simulink model "Load_Flow_V2"  (R2024a)
settings: Solver=ode23tb  StartTime=0.0  StopTime=0.3  RelTol=1e-4
undefined symbols (not defined in the file): Acid, D1, Delta, Lead
libraries: spsGroundLib x7, spsVoltageMeasurementLib x7, spsFourierLib x6, simulink x6, spsThreePhaseBreakerLib x4, spsThreePhaseTransformerTwoWindingsLib x3, spsThreePhaseParallelRLCLoadLib x3, spsThreePhaseSourceLib x2, spsThreePhaseFaultLib x2, spsBatteryLib x1, spsCurrentMeasurementLib x1, spsSeriesRLCBranchLib x1
settings Model: Creator=Sindid  LastModifiedBy=sindi
settings DataIOCC: SaveOutput=off

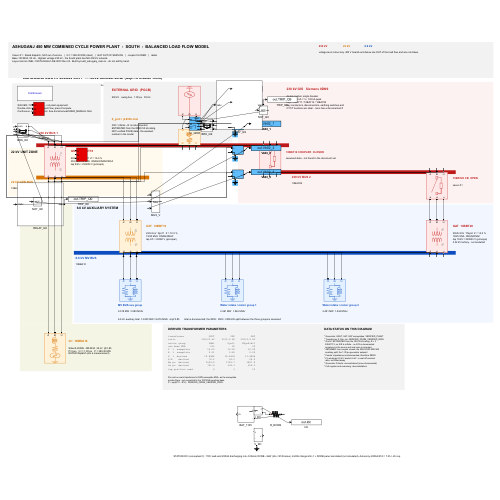
[thumbnail: Simulink's stored preview of the top-level diagram]
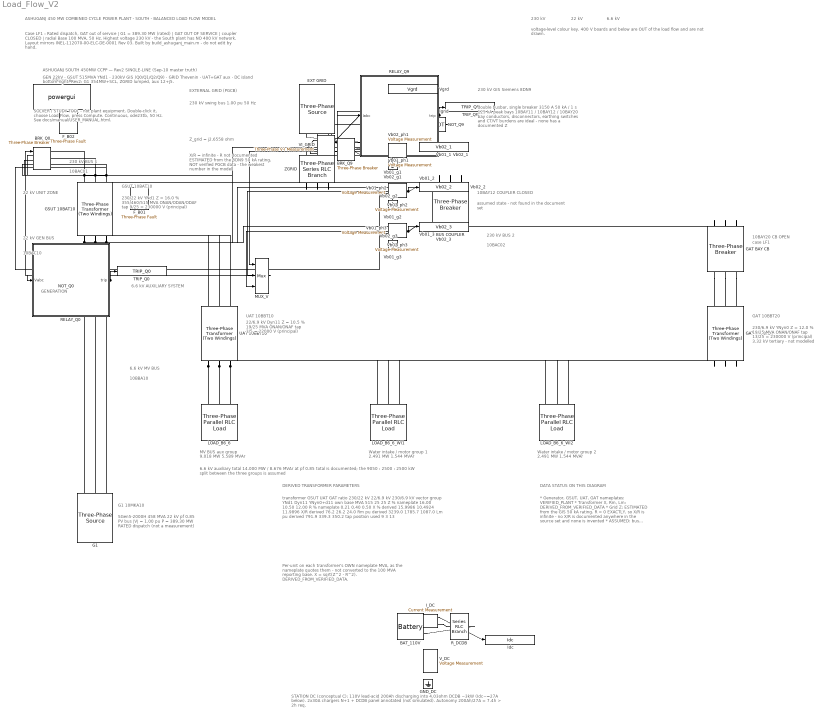
== system Load_Flow_V2 ==
  note: EXTERNAL GRID (PGCB)
  note: 230 kV swing bus 1.00 pu 50 Hz
  note: Z_grid = j2.6558 ohm
  note: X/R = infinite - R not documented
      | ESTIMATED from the 8DN9 50 kA rating,
      | NOT verified PGCB data - the weakest
      | number in the model
  note: GSUT 10BAT10
  note: 230/22 kV  YNd1  Z = 16.0 %
      | 355/460/515 MVA  ONAN/ODAN/ODAF
      | tap 9/25 = 230000 V (principal)
  note: 230 kV GIS Siemens 8DN9
  note: double busbar, single breaker
      | 3150 A  50 kA / 1 s  125 kA peak
      | bays 10BAY11 / 10BAY12 / 10BAY20
      | bay conductors, disconnectors, earthing switches and
      | CT/VT burdens are ideal - none has a documented Z
  note: 10BAY12 COUPLER CLOSED
  note: assumed state - not found in the document set
  note: 10BAY20 CB OPEN
  note: case LF1
  note: G1 10MKA10
  note: SGen5-2000H  458 MVA  22 kV  pf 0.85
      | PV bus   |V| = 1.00 pu   P = 389.30 MW
      | RATED dispatch (not a measurement)
  note: MV BUS aux group
  note: 9.018 MW 5.589 MVAr
  note: Water intake / motor group 1
  note: 2.491 MW 1.544 MVAr
  note: Water intake / motor group 2
  note: 2.491 MW 1.544 MVAr
  note: UAT 10BBT10
  note: 22/6.9 kV  Dyn11  Z = 10.5 %
      | 19/25 MVA  ONAN/ONAF
      | tap 3/5 = 22000 V (principal)
  note: GAT 10BBT20
  note: 230/6.9 kV  YNyn0  Z = 12.0 %
      | 19/25 MVA  ONAN/ONAF
      | tap 13/25 = 230000 V (principal)
      | 3.32 kV tertiary - not modelled
  note: 6.6 kV auxiliary total 14.000 MW / 8.676 MVAr at pf 0.85 total is documented; the 9050 : 2500 : 2500 kW split between the three groups is assumed
  note: 230 kV BUS 1
  note: 10BAC01
  note: 230 kV BUS 2
  note: 10BAC02
  note: 22 kV GEN BUS
  note: 10BAC10
  note: 6.6 kV MV BUS
  note: 10BBA10
  note: 22 kV UNIT ZONE
  note: 6.6 kV AUXILIARY SYSTEM
  note: GENERATION
  note: ASHUGANJ 450 MW COMBINED CYCLE POWER PLANT - SOUTH - BALANCED LOAD FLOW MODEL
  note: Case LF1 : Rated dispatch, GAT out of service   |   G1 = 389.30 MW (rated)   |   GAT OUT OF SERVICE   |   coupler CLOSED   |   radial
      | Base 100 MVA, 50 Hz.  Highest voltage 230 kV - the South plant has NO 400 kV network.
      | Layout mirrors INEL-112070-00-ELC-DE-0001 Rev 03.  Built by build_ashuganj_main.m - do not edit by hand.
  note: 230 kV
  note: 22 kV
  note: 6.6 kV
  note: voltage-level colour key. 400 V boards and below are OUT of the load flow and are not drawn.
  note: SOLVER / STUDY TOOL - not plant equipment.
      | Double-click it, choose Load Flow, press Compute.
      | Continuous, ode23tb, 50 Hz. See docs/manual/USER_MANUAL.html.
  note: DERIVED TRANSFORMER PARAMETERS
  note: transformer                 GSUT           UAT           GAT
      | ratio                  230/22 kV     22/6.9 kV    230/6.9 kV
      | vector group                YNd1         Dyn11     YNyn0+d11
      | own base MVA                 515            25            25
      | Z  %  nameplate            16.00         10.50         12.00
      | R  %  nameplate             0.21          0.40          0.50
      | X  %  derived            15.9986       10.4924       11.9896
      | X/R    derived              76.2          26.2          24.0
      | Rm pu  derived            3239.0        1785.7        1087.0
      | Lm pu  derived             791.9         339.3         350.2
      | tap position used              9             3            13
  note: Per-unit on each transformer's OWN nameplate MVA, as the nameplate
      | quotes them - not converted to the 100 MVA reporting base.
      | X = sqrt(Z^2 - R^2).  DERIVED_FROM_VERIFIED_DATA.
  note: DATA STATUS ON THIS DIAGRAM
  note: * Generator, GSUT, UAT, GAT nameplates: VERIFIED_PLANT
      | * Transformer X, Rm, Lm: DERIVED_FROM_VERIFIED_DATA
      | * Grid Z: ESTIMATED from the GIS 50 kA rating. R = 0
      |   EXACTLY, so X/R is infinite - no X/R is documented
      |   anywhere in the source set and none is invented
      | * ASSUMED: bus coupler closed, the 9050:2500:2500 kW
      |   auxiliary split, the 1.00 pu generator setpoint
      | * Feeder impedances undocumented, therefore ZERO
      | * LV windings 6.9 kV, loads 6.6 kV - a real off-nominal
      |   ratio, not tidied away
      | * Generator Q limits: unconstrained (none documented)
      | * Full register and reasoning: docs/validation/
  note: ASHUGANJ SOUTH 450MW CCPP — Rev2 SINGLE-LINE (Sep-10 master truth)
  note: GEN 22kV · GSUT 515MVA YNd1 · 230kV GIS (Q0/Q1/Q2/Q9) · GRID Thevenin · UAT+GAT aux · DC island bottom-right. Rev2: G1 354MW+SCL, ZGRID lumped, aux 12+j5.
  note: STATION DC (conceptual C): 110V lead-acid 200Ah discharging into 4.03ohm DCDB ~3kW (Idc~=27A below). 2x30A chargers N+1 + DCDB panel annotated (not simulated). Autonomy 200Ah/27A = 7.4h > 2h req.
  BAT_110V : spsBatteryLib/Battery  BatType=Lead-Acid  ShowTempParam=off  ThermalPreset=no  ShowAgeParam=off  NomV=110  NomQ=200  SOC=100  Batt_Tr=30  PresetModel=on  MaxQ=208.3333  MinV=82.5  FullV=119.7697  Dis_rate=40  R=0.0055  Normal_OP=62.0556  expZone="[111.9901     0.6666667]"  current=[6.5 13 32.5]  Units=Time  Tci=20  NomT=20  T2=-30  MaxQ2=4.8  FullV2=7.1  Normal_OP2=5.655  expZone2="[6.58           1]"  Rca=0.6  ti=2000  Dp=0  Neq0=0  Tsim=1e6  Ta1=25  Qeol=5.4*0.9  Reol=0.013333*1.2  Char_age=[2.3478, 3]  Dis_age=[2.3478, 10]  N1=1500  N2=10500  N3=1000  N4=1400  Ta2=45  N5=950
  BRK_Q0 : spsThreePhaseBreakerLib/Three-Phase Breaker  InitialState=closed  SwitchA=on  SwitchB=on  SwitchC=on  SwitchTimes="[1/60  5/60]"  External=on  BreakerResistance=0.01  SnubberResistance=1e6  SnubberCapacitance=inf  Measurements=None
  BRK_Q9 : spsThreePhaseBreakerLib/Three-Phase Breaker  InitialState=closed  SwitchA=on  SwitchB=on  SwitchC=on  SwitchTimes="[1/60  5/60]"  External=on  BreakerResistance=0.01  SnubberResistance=1e6  SnubberCapacitance=inf  Measurements=None
  BUS COUPLER : spsThreePhaseBreakerLib/Three-Phase Breaker  InitialState=closed  SwitchA=on  SwitchB=on  SwitchC=on  SwitchTimes=[1e6]  External=off  BreakerResistance=0.01  SnubberResistance=1e6  SnubberCapacitance=inf  Measurements=None
  EXT GRID : spsThreePhaseSourceLib/Three-Phase Source  InternalConnection=Yg  VoltagePhases=off  Voltage=230000  PhaseAngle=0  Voltage_phases=[25e3 25e3 25e3]/sqrt(3)  PhaseAngles_phases=[0 -120 +120]  Frequency=50  NonIdealSource=off  SpecifyImpedance=off  Resistance=0.8929  Inductance=16.58e-3  ShortCircuitLevel=100e6  BaseVoltage=230000  XRratio=7  BusType=swing  Pref=10e3  Qref=0  Prefabc=[10e3, 10e3, 10e3]  Qrefabc=[0, 0, 0]  Qmin=-inf  Qmax=inf
  F_B01 : spsThreePhaseFaultLib/Three-Phase Fault  InitialStates=0  FaultA=off  FaultB=off  FaultC=off  GroundFault=off  SwitchTimes=[0.05]  External=off  SwitchStatus=NaN  FaultResistance=1e-4  GroundResistance=1e-4  SnubberResistance=1e6  SnubberCapacitance=inf  Measurements=None
  F_B02 : spsThreePhaseFaultLib/Three-Phase Fault  InitialStates=0  FaultA=off  FaultB=off  FaultC=off  GroundFault=off  SwitchTimes=[0.05]  External=off  SwitchStatus=NaN  FaultResistance=1e-4  GroundResistance=1e-4  SnubberResistance=1e6  SnubberCapacitance=inf  Measurements=None
  G1 : spsThreePhaseSourceLib/Three-Phase Source  InternalConnection=Yg  VoltagePhases=off  Voltage=22000  PhaseAngle=0  Voltage_phases=[25e3 25e3 25e3]/sqrt(3)  PhaseAngles_phases=[0 -120 +120]  Frequency=50  NonIdealSource=on  SpecifyImpedance=on  Resistance=0.8929  Inductance=16.58e-3  ShortCircuitLevel=2.0374e9  BaseVoltage=22000  XRratio=266.9  BusType=PV  Pref=354e6  Qref=0  Prefabc=[10e3, 10e3, 10e3]  Qrefabc=[0, 0, 0]  Qmin=-inf  Qmax=inf
  GAT 10BBT20 : spsThreePhaseTransformerTwoWindingsLib/Three-Phase Transformer (Two Windings)  Winding1Connection=Yg  Winding2Connection=Yg  CoreType=Three single-phase transformers  SetSaturation=off  Hysteresis=off  DataFile='hysteresis'  SetInitialFlux=off  Measurements=None  UNITS=pu  NominalPower=[ 25000000 , 50 ]  Winding1=[ 230000 , 0.0025 , 0.0599478940414 ]  Winding2=[ 6900 , 0.0025 , 0.0599478940414 ]  Rm=1086.956522  Lm=350.2073842  L0=0.108  Saturation=[ 0,0 ; 0.0024,1.2 ; 1.0,1.52 ]  InitialFluxes=[ 0.8 , -0.8 , 0.7 ]  BreakLoop=off  DiscreteSolver=Trapezoidal iterative  DataType=off  TransfoNumber=1
  GAT BAY CB : spsThreePhaseBreakerLib/Three-Phase Breaker  InitialState=open  SwitchA=on  SwitchB=on  SwitchC=on  SwitchTimes=[1e6]  External=off  BreakerResistance=0.01  SnubberResistance=1e6  SnubberCapacitance=inf  Measurements=None
  GND_DC : spsGroundLib/Ground  LConnTagsString=a
  GSUT 10BAT10 : spsThreePhaseTransformerTwoWindingsLib/Three-Phase Transformer (Two Windings)  Winding1Connection=Yg  Winding2Connection=Delta (D1)  CoreType=Three single-phase transformers  SetSaturation=off  Hysteresis=off  DataFile='hysteresis'  SetInitialFlux=off  Measurements=None  UNITS=pu  NominalPower=[ 515000000 , 50 ]  Winding1=[ 230000 , 0.0008855 , 0.083145 ]  Winding2=[ 22000 , 0.0008855 , 0.083145 ]  Rm=3316.5  Lm=791.8867922  L0=0.1663  Saturation=[ 0,0 ; 0.0024,1.2 ; 1.0,1.52 ]  InitialFluxes=[ 0.8 , -0.8 , 0.7 ]  BreakLoop=off  DiscreteSolver=Trapezoidal iterative  DataType=off  TransfoNumber=1
  I_DC : spsCurrentMeasurementLib/Current Measurement  PhasorSimulation=off  OutputType=Complex  PSBequivalent=0
  Idc : ToWorkspace  VariableName=Idc  SaveFormat=Structure With Time  SampleTime=5e-5
  Igrid : ToWorkspace  VariableName=Igrid  SaveFormat=Structure With Time  SampleTime=5e-5
  LOAD_B6_6 : spsThreePhaseParallelRLCLoadLib/Three-Phase Parallel RLC Load  LConnTagsString=A|B|C  Configuration=Y (grounded)  NominalVoltage=6600  Vabc=[1e3 1e3 1e3]  Vabcp=[1e3 1e3 1e3]  NominalFrequency=50  UnbalancedPower=off  ActivePower=12e6  InductivePower=5e6  CapacitivePower=0  Pabc=[10e3 9e3 11e3]  QLabc=[100 90 110]  QCabc=[100 90 110]  Pabcp=[10e3 9e3 11e3]  QLabcp=[100 90 110]  QCabcp=[100 90 110]  Measurements=None  LoadType=constant PQ
  LOAD_B6_6_WI1 : spsThreePhaseParallelRLCLoadLib/Three-Phase Parallel RLC Load  LConnTagsString=A|B|C  Configuration=Y (grounded)  NominalVoltage=6600  Vabc=[1e3 1e3 1e3]  Vabcp=[1e3 1e3 1e3]  NominalFrequency=50  UnbalancedPower=off  ActivePower=1  InductivePower=1  CapacitivePower=0  Pabc=[10e3 9e3 11e3]  QLabc=[100 90 110]  QCabc=[100 90 110]  Pabcp=[10e3 9e3 11e3]  QLabcp=[100 90 110]  QCabcp=[100 90 110]  Measurements=None  LoadType=constant PQ
  LOAD_B6_6_WI2 : spsThreePhaseParallelRLCLoadLib/Three-Phase Parallel RLC Load  LConnTagsString=A|B|C  Configuration=Y (grounded)  NominalVoltage=6600  Vabc=[1e3 1e3 1e3]  Vabcp=[1e3 1e3 1e3]  NominalFrequency=50  UnbalancedPower=off  ActivePower=1  InductivePower=1  CapacitivePower=0  Pabc=[10e3 9e3 11e3]  QLabc=[100 90 110]  QCabc=[100 90 110]  Pabcp=[10e3 9e3 11e3]  QLabcp=[100 90 110]  QCabcp=[100 90 110]  Measurements=None  LoadType=constant PQ
  MUX_V : Mux  Inputs=3
  NOT_Q0 : Logic  Operator=NOT  AllPortsSameDT=off  OutDataTypeStr=boolean
  NOT_Q9 : Logic  Operator=NOT  AllPortsSameDT=off  OutDataTypeStr=boolean
  RELAY_Q0 : Subsystem
  RELAY_Q9 : Subsystem
  R_DCDB : spsSeriesRLCBranchLib/Series RLC Branch  LConnTagsString=__new0  RConnTagsString=__new0  BranchType=R  Resistance=4.033  Inductance=1e-3  SetiL0=off  InitialCurrent=0  Capacitance=1e-6  Setx0=off  InitialVoltage=0  Measurements=None
  TRIP_Q0 : ToWorkspace  VariableName=TRIP_Q0  SaveFormat=Structure With Time  SampleTime=5e-5
  TRIP_Q9 : ToWorkspace  VariableName=TRIP_Q9  SaveFormat=Structure With Time  SampleTime=5e-5
  UAT 10BBT10 : spsThreePhaseTransformerTwoWindingsLib/Three-Phase Transformer (Two Windings)  Winding1Connection=Delta (D1)  Winding2Connection=Yg  CoreType=Three single-phase transformers  SetSaturation=off  Hysteresis=off  DataFile='hysteresis'  SetInitialFlux=off  Measurements=None  UNITS=pu  NominalPower=[ 25000000 , 50 ]  Winding1=[ 22000 , 0.002 , 0.0524618909305 ]  Winding2=[ 6900 , 0.002 , 0.0524618909305 ]  Rm=1785.714286  Lm=339.2970532  L0=0.093  Saturation=[ 0,0 ; 0.0024,1.2 ; 1.0,1.52 ]  InitialFluxes=[ 0.8 , -0.8 , 0.7 ]  BreakLoop=off  DiscreteSolver=Trapezoidal iterative  DataType=off  TransfoNumber=1
  VI_GRID : spsThreePhaseVIMeasurementLib/Three-Phase V-I Measurement  VoltageMeasurement=phase-to-ground  SetLabelV=off  LabelV=Vabc  Vpu=off  VpuLL=off  CurrentMeasurement=yes  SetLabelI=off  LabelI=Iabc  Ipu=off  Pbase=100e6  Vbase=500e3  OutputType=Complex  PhasorSimulation=off  PSBequivalent=0
  V_DC : spsVoltageMeasurementLib/Voltage Measurement  PhasorSimulation=off  OutputType=Complex  PSBequivalent=0
  Vb01_1 : ToWorkspace  VariableName=Vb01_1  SaveFormat=Structure With Time  SampleTime=5e-5
  Vb01_2 : ToWorkspace  VariableName=Vb01_2  SaveFormat=Structure With Time  SampleTime=5e-5
  Vb01_3 : ToWorkspace  VariableName=Vb01_3  SaveFormat=Structure With Time  SampleTime=5e-5
  Vb01_g1 : spsGroundLib/Ground  LConnTagsString=a
  Vb01_g2 : spsGroundLib/Ground  LConnTagsString=a
  Vb01_g3 : spsGroundLib/Ground  LConnTagsString=a
  Vb01_ph1 : spsVoltageMeasurementLib/Voltage Measurement  PhasorSimulation=off  OutputType=Complex  PSBequivalent=0
  Vb01_ph2 : spsVoltageMeasurementLib/Voltage Measurement  PhasorSimulation=off  OutputType=Complex  PSBequivalent=0
  Vb01_ph3 : spsVoltageMeasurementLib/Voltage Measurement  PhasorSimulation=off  OutputType=Complex  PSBequivalent=0
  Vb02_1 : ToWorkspace  VariableName=Vb02_1  SaveFormat=Structure With Time  SampleTime=5e-5
  Vb02_2 : ToWorkspace  VariableName=Vb02_2  SaveFormat=Structure With Time  SampleTime=5e-5
  Vb02_3 : ToWorkspace  VariableName=Vb02_3  SaveFormat=Structure With Time  SampleTime=5e-5
  Vb02_g1 : spsGroundLib/Ground  LConnTagsString=a
  Vb02_g2 : spsGroundLib/Ground  LConnTagsString=a
  Vb02_g3 : spsGroundLib/Ground  LConnTagsString=a
  Vb02_ph1 : spsVoltageMeasurementLib/Voltage Measurement  PhasorSimulation=off  OutputType=Complex  PSBequivalent=0
  Vb02_ph2 : spsVoltageMeasurementLib/Voltage Measurement  PhasorSimulation=off  OutputType=Complex  PSBequivalent=0
  Vb02_ph3 : spsVoltageMeasurementLib/Voltage Measurement  PhasorSimulation=off  OutputType=Complex  PSBequivalent=0
  Vgrd : ToWorkspace  VariableName=Vgrd  SaveFormat=Structure With Time  SampleTime=5e-5
  ZGRID : spsThreePhaseSeriesRLCBranchLib/Three-Phase Series RLC Branch  LConnTagsString=A|B|C  RConnTagsString=A|B|C  BranchType=RL  Resistance=0.296  Inductance=9.747e-3  Capacitance=1e-6  Measurements=None
  powergui : sps_lib/powergui  Priority=1  SimulationMode=Continuous  SampleTime=50e-6  frequency=50  Iterations=50  frequencyindice=50  Pbase=100000000  ErrMax=1e-4  UnitsV=kV  UnitsW=MW  buscounter=0  FunctionMessages=off  echomessages=off  EnableUseOfTLC=off  CurrentSourceSwitches=off  DisableSnubberDevices=off  DisableRonSwitches=off  DisableVfSwitches=off  DisplayEquations=off  AutomaticDiscreteSolvers=off  SolverType=Tustin/Backward Euler (TBE)  Interpol=off  ExternalGateDelay=off  methode=off  Ts=100  x0status=blocks  SPID=on  SwTol=0  HookPort=off  NonlinearTolerance=1e-4  nMaxIteration=100  ContinueOnMaxIteration=off  RestoreLinks=warning  ResistiveCurrentMeasurement=off  Frange=[0:2:500]  Ylog=off  Xlog=on  ShowGrid=off  save=off  variable=ZData  structure=0  ZoomFFT=off  StartTime=0.0  cycles=1  DisplayStyle=1  fundamental=60  FreqAxis=off  MaxFrequency=1000  frequencyindicesteady=1  RmsSteady=1  display=off
  wires:
  VI_GRID/1 -> Vgrd/1
  VI_GRID/2 -> Igrid/1, RELAY_Q9/1(Iabc)
  Vb01_ph1/1 -> Vb01_1/1
  Vb01_ph2/1 -> Vb01_2/1
  Vb01_ph3/1 -> Vb01_3/1
  Vb02_ph1/1 -> Vb02_1/1, MUX_V/1
  Vb02_ph2/1 -> Vb02_2/1, MUX_V/2
  Vb02_ph3/1 -> Vb02_3/1, MUX_V/3
  I_DC/1 -> Idc/1
  RELAY_Q9/1(trip) -> NOT_Q9/1, TRIP_Q9/1
  NOT_Q9/1 -> BRK_Q9/1
  MUX_V/1 -> RELAY_Q0/1(Vabc)
  RELAY_Q0/1(trip) -> NOT_Q0/1, TRIP_Q0/1
  NOT_Q0/1 -> BRK_Q0/1
  connections:
  GAT BAY CB/LConn1 -- BUS COUPLER/RConn1
  GAT BAY CB/LConn2 -- BUS COUPLER/RConn2
  GAT BAY CB/LConn3 -- BUS COUPLER/RConn3
  GAT 10BBT20/RConn1 -- LOAD_B6_6/LConn1 -- LOAD_B6_6_WI1/LConn1 -- UAT 10BBT10/RConn1 -- LOAD_B6_6_WI2/LConn1
  GAT 10BBT20/RConn2 -- LOAD_B6_6/LConn2 -- LOAD_B6_6_WI1/LConn2 -- UAT 10BBT10/RConn2 -- LOAD_B6_6_WI2/LConn2
  GAT 10BBT20/RConn3 -- LOAD_B6_6/LConn3 -- LOAD_B6_6_WI1/LConn3 -- UAT 10BBT10/RConn3 -- LOAD_B6_6_WI2/LConn3
  ZGRID/LConn1 -- BUS COUPLER/LConn1 -- BRK_Q0/RConn1 -- Vb02_ph1/LConn1
  ZGRID/LConn2 -- BUS COUPLER/LConn2 -- BRK_Q0/RConn2 -- Vb02_ph2/LConn1
  ZGRID/LConn3 -- BUS COUPLER/LConn3 -- BRK_Q0/RConn3 -- Vb02_ph3/LConn1
  G1/RConn1 -- UAT 10BBT10/LConn1 -- GSUT 10BAT10/RConn1 -- Vb01_ph1/LConn1
  G1/RConn2 -- UAT 10BBT10/LConn2 -- GSUT 10BAT10/RConn2 -- Vb01_ph2/LConn1
  G1/RConn3 -- UAT 10BBT10/LConn3 -- GSUT 10BAT10/RConn3 -- Vb01_ph3/LConn1
  GAT BAY CB/RConn1 -- GAT 10BBT20/LConn1
  GAT BAY CB/RConn2 -- GAT 10BBT20/LConn2
  GAT BAY CB/RConn3 -- GAT 10BBT20/LConn3
  ZGRID/RConn1 -- VI_GRID/LConn1
  ZGRID/RConn2 -- VI_GRID/LConn2
  ZGRID/RConn3 -- VI_GRID/LConn3
  Vb01_ph1/LConn2 -- Vb01_g1/LConn1
  Vb01_ph2/LConn2 -- Vb01_g2/LConn1
  Vb01_ph3/LConn2 -- Vb01_g3/LConn1
  Vb02_ph1/LConn2 -- Vb02_g1/LConn1
  Vb02_ph2/LConn2 -- Vb02_g2/LConn1
  Vb02_ph3/LConn2 -- Vb02_g3/LConn1
  BAT_110V/LConn1 -- I_DC/LConn1
  I_DC/RConn1 -- R_DCDB/LConn1
  R_DCDB/RConn1 -- BAT_110V/LConn2
  VI_GRID/RConn1 -- BRK_Q9/LConn1
  BRK_Q9/RConn1 -- EXT GRID/RConn1
  VI_GRID/RConn2 -- BRK_Q9/LConn2
  BRK_Q9/RConn2 -- EXT GRID/RConn2
  VI_GRID/RConn3 -- BRK_Q9/LConn3
  BRK_Q9/RConn3 -- EXT GRID/RConn3
  GSUT 10BAT10/LConn1 -- BRK_Q0/LConn1
  GSUT 10BAT10/LConn2 -- BRK_Q0/LConn2
  GSUT 10BAT10/LConn3 -- BRK_Q0/LConn3

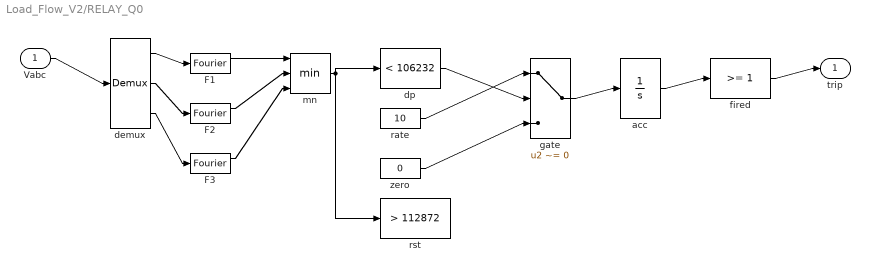
== system Load_Flow_V2/RELAY_Q0 ==
  Vabc : Inport
  F1 : spsFourierLib/Fourier  Freq=50  n=1  InInit=[0, 0]  Ts=0
  F2 : spsFourierLib/Fourier  Freq=50  n=1  InInit=[0, 0]  Ts=0
  F3 : spsFourierLib/Fourier  Freq=50  n=1  InInit=[0, 0]  Ts=0
  acc : Integrator
  demux : Demux  Outputs=3
  dp : simulink/Logic and Bit Operations/Compare To Constant  relop=<  const=106232  OutDataTypeStr=boolean
  fired : simulink/Logic and Bit Operations/Compare To Constant  relop=>=  const=1  OutDataTypeStr=boolean
  gate : Switch  Criteria=u2 ~= 0
  mn : MinMax  Inputs=3
  rate : Constant  Value=10
  rst : simulink/Logic and Bit Operations/Compare To Constant  relop=>  const=112872  OutDataTypeStr=boolean
  zero : Constant  Value=0
  trip : Outport
  wires:
  Vabc/1 -> demux/1
  demux/1 -> F1/1
  F1/1 -> mn/1
  demux/2 -> F2/1
  F2/1 -> mn/2
  demux/3 -> F3/1
  F3/1 -> mn/3
  mn/1 -> dp/1, rst/1
  rate/1 -> gate/1
  dp/1 -> gate/2
  zero/1 -> gate/3
  gate/1 -> acc/1
  acc/1 -> fired/1
  fired/1 -> trip/1

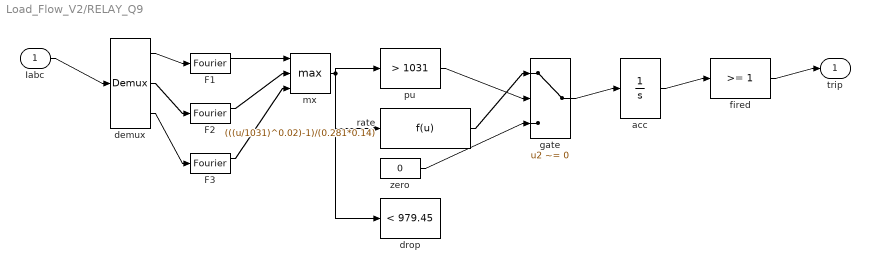
== system Load_Flow_V2/RELAY_Q9 ==
  Iabc : Inport
  F1 : spsFourierLib/Fourier  Freq=50  n=1  InInit=[0, 0]  Ts=0
  F2 : spsFourierLib/Fourier  Freq=50  n=1  InInit=[0, 0]  Ts=0
  F3 : spsFourierLib/Fourier  Freq=50  n=1  InInit=[0, 0]  Ts=0
  acc : Integrator
  demux : Demux  Outputs=3
  drop : simulink/Logic and Bit Operations/Compare To Constant  relop=<  const=979.45  OutDataTypeStr=boolean
  fired : simulink/Logic and Bit Operations/Compare To Constant  relop=>=  const=1  OutDataTypeStr=boolean
  gate : Switch  Criteria=u2 ~= 0
  mx : MinMax  Function=max  Inputs=3
  pu : simulink/Logic and Bit Operations/Compare To Constant  relop=>  const=1031  OutDataTypeStr=boolean
  rate : Fcn  Expr=(((u/1031)^0.02)-1)/(0.281*0.14)
  zero : Constant  Value=0
  trip : Outport
  wires:
  Iabc/1 -> demux/1
  demux/1 -> F1/1
  F1/1 -> mx/1
  demux/2 -> F2/1
  F2/1 -> mx/2
  demux/3 -> F3/1
  F3/1 -> mx/3
  mx/1 -> pu/1, rate/1, drop/1
  rate/1 -> gate/1
  pu/1 -> gate/2
  zero/1 -> gate/3
  gate/1 -> acc/1
  acc/1 -> fired/1
  fired/1 -> trip/1
